simulink model "test"  (R2021b)
settings: Solver=VariableStepAuto  StartTime=0.0  StopTime=0.01  RelTol=1e-3
libraries: spsSeriesRLCBranchLib x5, spsControlledVoltageSourceLib x1, spsGroundLib x1, spsMultimeterLib x1, eeSinusoidalMeasurementV2 x1, spsTriangleGeneratorLib x1, spspowerguiLib x1
settings Model: Creator=NicholasYe  LastModifiedBy=NicholasYe
settings DataIOCC: ReturnWorkspaceOutputs=off

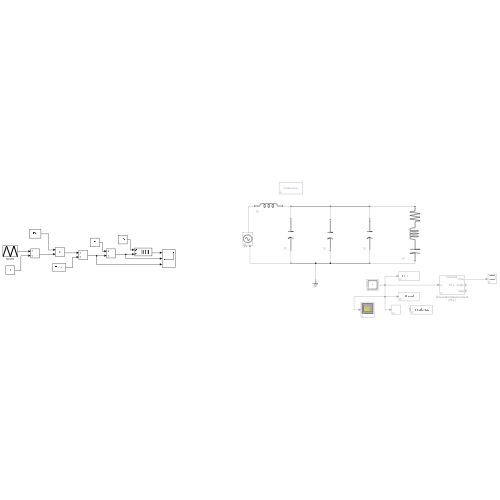
[thumbnail: Simulink's stored preview of the top-level diagram]
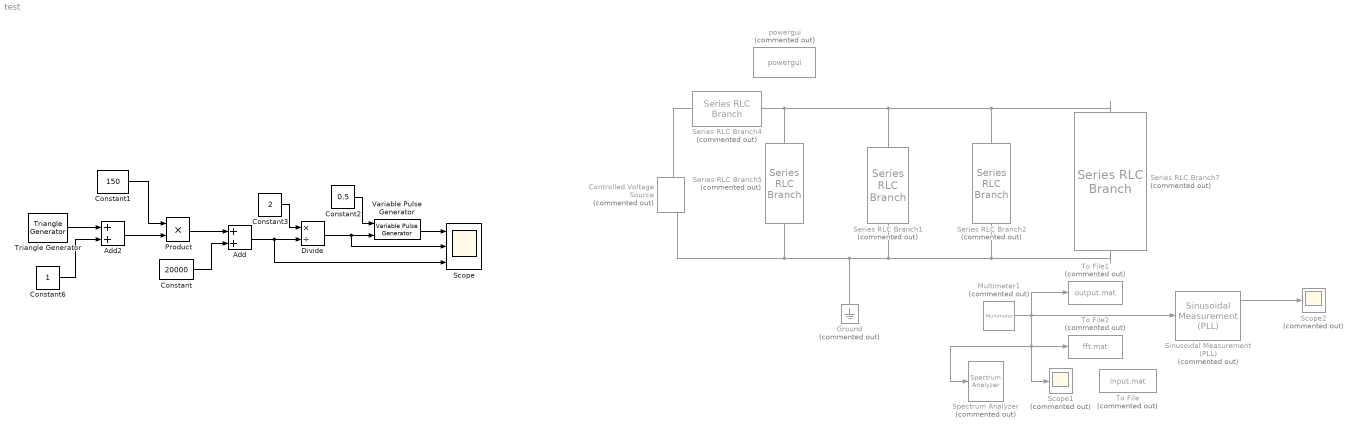
== system test ==
  Add : Sum
  Add2 : Sum
  Constant : Constant  Value=20000
  Constant1 : Constant  Value=150
  Constant2 : Constant  Value=0.5
  Constant3 : Constant  Value=2
  Constant6 : Constant
  Controlled Voltage Source : spsControlledVoltageSourceLib/Controlled Voltage Source  Commented=on  Initialize=on  Source_Type=AC  Amplitude=100  Phase=0  Frequency=20000  Measurements=Voltage
  Divide : Product  Inputs=*/
  Ground : spsGroundLib/Ground  Commented=on  LConnTagsString=a
  Multimeter1 : spsMultimeterLib/Multimeter  Commented=on  PhasorSimulation=off  OutputType=Complex  sel=1  L=2  Gain=1  yselected={'Ub: Series RLC Branch2'};  PSBOutputType=1  PSBequivalent=0  AxesSetting=[0,0.1,-100,100]  Display=0  SavedBlockNames=-11
  Product : Product
  Scope : Scope  NumInputPorts=3
  Scope1 : Scope  Commented=on
  Scope2 : Scope  Commented=on
  Series RLC Branch1 : spsSeriesRLCBranchLib/Series RLC Branch  Commented=on  LConnTagsString=__new0  RConnTagsString=__new0  BranchType=C  Resistance=0  Inductance=inf  SetiL0=off  InitialCurrent=0  Capacitance=6.8e-9  Setx0=off  InitialVoltage=0  Measurements=None
  Series RLC Branch2 : spsSeriesRLCBranchLib/Series RLC Branch  Commented=on  LConnTagsString=__new0  RConnTagsString=__new0  BranchType=C  Resistance=0  Inductance=inf  SetiL0=off  InitialCurrent=0  Capacitance=12.023e-9  Setx0=off  InitialVoltage=0  Measurements=Branch voltage
  Series RLC Branch4 : spsSeriesRLCBranchLib/Series RLC Branch  Commented=on  LConnTagsString=__new0  RConnTagsString=__new0  BranchType=L  Resistance=0  Inductance=0.00134  SetiL0=off  InitialCurrent=0  Capacitance=inf  Setx0=off  InitialVoltage=0  Measurements=None
  Series RLC Branch5 : spsSeriesRLCBranchLib/Series RLC Branch  Commented=on  LConnTagsString=__new0  RConnTagsString=__new0  BranchType=C  Resistance=0  Inductance=inf  SetiL0=off  InitialCurrent=0  Capacitance=6.8e-9  Setx0=off  InitialVoltage=0  Measurements=None
  Series RLC Branch7 : spsSeriesRLCBranchLib/Series RLC Branch  Commented=on  LConnTagsString=__new0  RConnTagsString=__new0  BranchType=RLC  Resistance=124.09  Inductance=1.463  SetiL0=off  InitialCurrent=0  Capacitance=42.528e-12  Setx0=off  InitialVoltage=0  Measurements=None
  Sinusoidal Measurement (PLL) : eeSinusoidalMeasurementV2/Sinusoidal Measurement (PLL)  Commented=on  Ki_PD=1000  Kp_LF=400  Ki_LF=20000  F0=60  Theta0=0  Mag0=1  Ts=-1
      settings: SourceProductBaseCode=PS
  Spectrum Analyzer : SpectrumAnalyzer  Commented=on
  To File : ToFile  Commented=on  Filename=input.mat  MatrixName=input
  To File1 : ToFile  Commented=on  Filename=output.mat  MatrixName=output
  To File2 : ToFile  Commented=on  Filename=fft.mat  MatrixName=output
  Triangle Generator : spsTriangleGeneratorLib/Triangle Generator  Freq=500  Phase=0  Ts=0
      settings: AttributesFormatString=%<Freq>Hz
  Variable Pulse Generator : VariablePulseGenerator  SampleTime=0.1
  powergui : spspowerguiLib/powergui  Priority=1  Commented=on  SimulationMode=Continuous  SampleTime=1e-8  frequency=60  Iterations=50  frequencyindice=20000  Pbase=100e6  ErrMax=1e-4  UnitsV=kV  UnitsW=MW  buscounter=0  FunctionMessages=off  echomessages=off  EnableUseOfTLC=off  CurrentSourceSwitches=off  DisableSnubberDevices=off  DisableRonSwitches=off  DisableVfSwitches=off  DisplayEquations=off  AutomaticDiscreteSolvers=off  SolverType=Tustin/Backward Euler (TBE)  Interpol=off  ExternalGateDelay=off  methode=off  Ts=100  x0status=blocks  SPID=on  SwTol=0  HookPort=off  NonlinearTolerance=1e-4  nMaxIteration=100  ContinueOnMaxIteration=off  RestoreLinks=warning  ResistiveCurrentMeasurement=off  Frange=[0:2:500]  Ylog=off  Xlog=on  ShowGrid=off  save=off  variable=ZData  structure=0  ZoomFFT=off  StartTime=0.0  cycles=1  DisplayStyle=1  fundamental=60  FreqAxis=off  MaxFrequency=1000  frequencyindicesteady=1  RmsSteady=1  display=off
  wires:
  Constant1/1 -> Product/1
  Product/1 -> Add/1
  Constant/1 -> Add/2
  Constant2/1 -> Variable Pulse Generator/1
  Constant3/1 -> Divide/1
  Multimeter1/1 -> To File2/1, Scope1/1, Spectrum Analyzer/1, To File1/1, Sinusoidal Measurement (PLL)/1
  Add/1 -> Scope/3, Divide/2
  Triangle Generator/1 -> Add2/1
  Add2/1 -> Product/2
  Constant6/1 -> Add2/2
  Sinusoidal Measurement (PLL)/1 -> Scope2/1
  Variable Pulse Generator/1 -> Scope/1
  Divide/1 -> Scope/2, Variable Pulse Generator/2
  connections:
  Controlled Voltage Source/RConn1 -- Series RLC Branch4/LConn1
  Series RLC Branch7/LConn1 -- Series RLC Branch2/LConn1 -- Series RLC Branch1/LConn1 -- Series RLC Branch5/LConn1 -- Series RLC Branch4/RConn1
  Series RLC Branch7/RConn1 -- Series RLC Branch2/RConn1 -- Series RLC Branch1/RConn1 -- Ground/LConn1 -- Series RLC Branch5/RConn1 -- Controlled Voltage Source/LConn1
